simulink model "lab_3"  (R2020b)
settings: Solver=VariableStepAuto  StartTime=0.0  StopTime=100  RelTol=1e-3
InitFcn:
  | A = [0 1; -8 -4];
  | b = [3; 2];
  | C = [1 0];
  | W = [4 5; 5 7];
  | V = 45;
  | G= eye(2);
  | 
  | syms p11 p12 p22;
  | P = [p11 p12; p12 p22];
  | egn1 = A*P + P*A' + G*W*G' - P*C'*inv(V)*C*P == 0;
  | solution = solve([egn1], [p11, p12, p22]);
  | p11_sol = double(solution.p11)
  | p12_sol = double(solution.p12)
  | p22_sol = double(solution.p22)
  | 
  | Pp = [p11_sol(1) p12_sol(1); p12_sol(1) p22_sol(1)];
  | L = Pp*C'*inv(V);
libraries: simulink x1
settings Model: Creator=Eugene  LastModifiedBy=Eugene

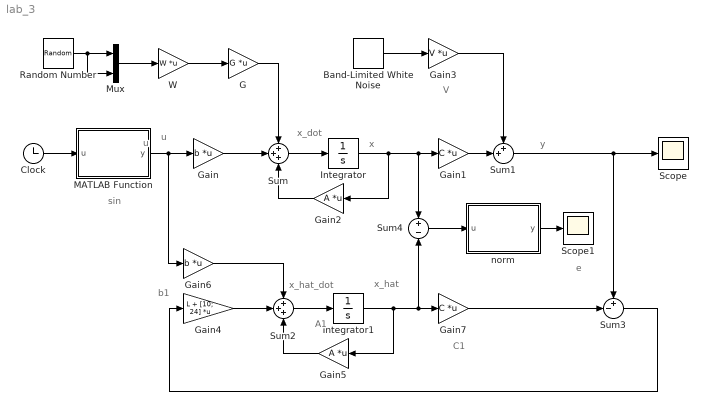
== system lab_3 ==
  note: e
  note: V
  note: A1
  note: C1
  note: b1
  note: y
  note: u
  note: sin
  note: x
  note: x_dot
  note: u
  note: x_hat
  note: x_hat_dot
  Band-Limited White Noise : simulink/Sources/Band-Limited White Noise  Cov=[0.1]  Ts=0.1  seed=[23341]
  Clock : Clock
  G : Gain  Gain=G  Multiplication=Matrix(K*u)
  Gain : Gain  Gain=b  Multiplication=Matrix(K*u)
  Gain1 : Gain  Gain=C  Multiplication=Matrix(K*u)
  Gain2 : Gain  Gain=A  Multiplication=Matrix(K*u)
  Gain3 : Gain  Gain=V  Multiplication=Matrix(K*u)
  Gain4 : Gain  Gain=L + [10; 24]  Multiplication=Matrix(K*u)
  Gain5 : Gain  Gain=A  Multiplication=Matrix(K*u)
  Gain6 : Gain  Gain=b  Multiplication=Matrix(K*u)
  Gain7 : Gain  Gain=C  Multiplication=Matrix(K*u)
  Integrator : Integrator  InitialCondition=[1; 0]
  Integrator1 : Integrator  InitialCondition=[0; 0]
  MATLAB Function : MATLAB Function  TreatAsAtomicUnit=on
  Mux : Mux  Inputs=2
  Random Number : RandomNumber  SampleTime=0.1
  Scope : Scope
  Scope1 : Scope
  Sum : Sum  Inputs=+++
  Sum1 : Sum  Inputs=++|
  Sum2 : Sum  Inputs=+++
  Sum3 : Sum  Inputs=+-|
  Sum4 : Sum  Inputs=+-
  W : Gain  Gain=W  Multiplication=Matrix(K*u)
  norm : MATLAB Function  TreatAsAtomicUnit=on
  wires:
  Sum/1 -> Integrator/1
  Integrator/1 -> Gain1/1, Sum4/1, Gain2/1
  Random Number/1 -> Mux/2, Mux/1
  Gain2/1 -> Sum/3
  Gain/1 -> Sum/2
  G/1 -> Sum/1
  Clock/1 -> MATLAB Function/1(u)
  MATLAB Function/1(y) -> Gain6/1, Gain/1
  Gain1/1 -> Sum1/2
  Band-Limited White Noise/1 -> Gain3/1
  Gain3/1 -> Sum1/1
  Sum1/1 -> Scope/1, Sum3/1
  Sum2/1 -> Integrator1/1
  Gain6/1 -> Sum2/1
  Gain5/1 -> Sum2/3
  Integrator1/1 -> Sum4/2, Gain7/1, Gain5/1
  Gain4/1 -> Sum2/2
  Gain7/1 -> Sum3/2
  Sum3/1 -> Gain4/1
  norm/1(y) -> Scope1/1
  Sum4/1 -> norm/1(u)
  W/1 -> G/1
  Mux/1 -> W/1

== matlab function lab_3/MATLAB Function ==
  data: u input; y output
function y = fcn(u)

y = sin(u);

== matlab function lab_3/norm ==
  data: u input; y output
function y = fcn(u)

y = norm(u);
